simulink subsystem "model_inductance_sensitivity_distance"  (R2024a)
settings: Solver=VariableStepAuto  StartTime=0.0  StopTime=10.0  RelTol=1e-3
values from neighbouring files (symbols this model uses):
  a = 1 / 0.0058231    (= 171.729834624)    [maglev_parameters.m]
  d = 0.20    (= 0.2)    [maglev_parameters.m]
  Ld = 0.017521    [maglev_parameters.m]
settings Model: Creator=Bocchio  LastModifiedBy=Bocchio

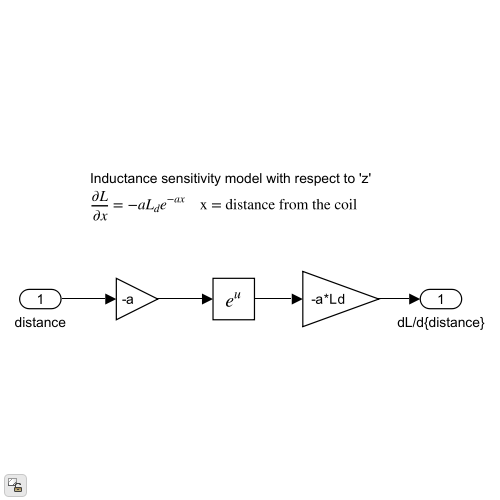
[thumbnail: Simulink's stored preview of the top-level diagram]
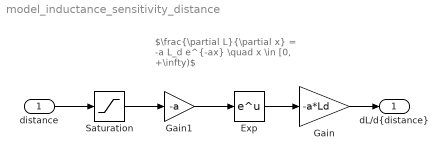
== system model_inductance_sensitivity_distance ==
  note: $\frac{\partial L}{\partial x} = -a L_d e^{-ax} \quad x \in [0, +\infty)$
  distance : Inport
  Exp : Math
  Gain : Gain  Gain=-a*Ld
  Gain1 : Gain  Gain=-a
  Saturation : Saturate  UpperLimit=d  LowerLimit=0
  "dL/d{distance}" : Outport
  wires:
  distance/1 -> Saturation/1
  Saturation/1 -> Gain1/1
  Gain1/1 -> Exp/1
  Exp/1 -> Gain/1
  Gain/1 -> "dL/d{distance}"/1
